simulink model "SetData"  (R2015a)
settings: configuration reference "config_cosim" (kept outside this file)
PreLoadFcn:
  | load config_cosim
model workspace (MAT data in the model file):
  Target.Ind = [1 0 1 0 0 0 1 0]
  Target.FSC = [1 0 1 0 0 0 4 0]
  Target.DD = [1  0; 0  0; 0  1; 0  0; 0  0; 0  0; 0  1; 0  0]
  Target.Ind0 = 0
  cmd_asn_cfm1 = [1 0 1 0 0 0 1 0]
  t_delta = 1
settings Model: CovModelRefEnable=off  Creator=zhang  LastModifiedBy=yrzhang
settings ConfigSetRef: SourceLocation=Base Workspace

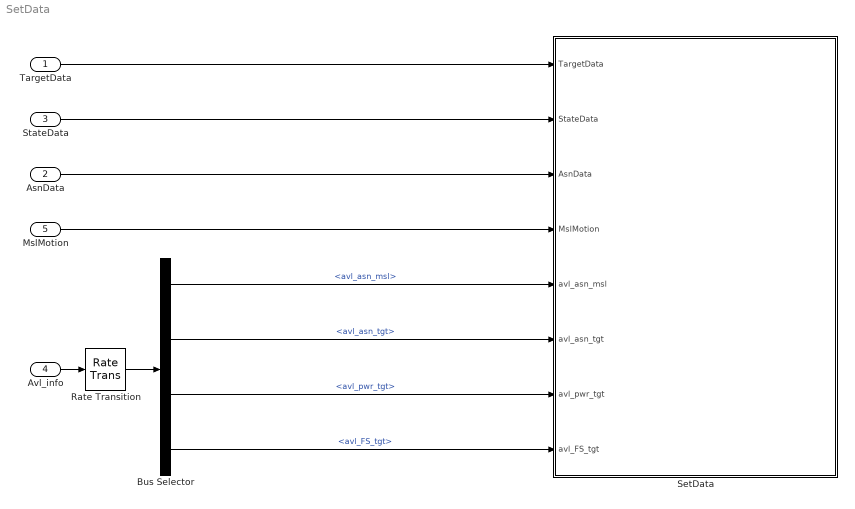
== system SetData ==
  TargetData : Inport  OutDataTypeStr=Bus: TgtDataLDBusObject
  AsnData : Inport  Port=2  OutDataTypeStr=double
  StateData : Inport  Port=3  OutDataTypeStr=Bus:StateBusObject
  Avl_info : Inport  Port=4  OutDataTypeStr=Bus: AvlBusObject
  MslMotion : Inport  Port=5  OutDataTypeStr=Bus: MslDataBusObject
  Bus Selector : BusSelector  OutputSignals=avl_asn_msl,avl_asn_tgt,avl_pwr_tgt,avl_FS_tgt
  Rate Transition : RateTransition
  SetData : Stateflow chart  TreatAsAtomicUnit=on
  wires:
  TargetData/1 -> SetData/1(TargetData)
  StateData/1 -> SetData/2(StateData)
  Avl_info/1 -> Rate Transition/1
  Bus Selector/1 -> SetData/5(avl_asn_msl)  "<avl_asn_msl>"
  Bus Selector/2 -> SetData/6(avl_asn_tgt)  "<avl_asn_tgt>"
  Bus Selector/3 -> SetData/7(avl_pwr_tgt)  "<avl_pwr_tgt>"
  Bus Selector/4 -> SetData/8(avl_FS_tgt)  "<avl_FS_tgt>"
  Rate Transition/1 -> Bus Selector/1
  AsnData/1 -> SetData/3(AsnData)
  MslMotion/1 -> SetData/4(MslMotion)

== stateflow chart SetData/SetData ==
  state Init
    entry,during: coder.extrinsic('display_control');
    h = display_control('SetData',TargetData,AsnData,MslMotion,StateData);
    %h = display_control('EnableUIControl',avl_asn_msl2,avl_pwr_tgt,avl_FS_tgt);
  data: TargetData input Bus: TgtDataLDBusObject size=1; StateData input Bus: StateBusObject size=1; AsnData input size=[8 2]; MslMotion input Bus: MslDataBusObject size=1; avl_asn_msl input size=8; avl_asn_tgt input size=8; avl_pwr_tgt input size=8; avl_FS_tgt input size=8; h local double
